simulink model "COM_test_gumstix"  (Simulink 8.6)
settings: Solver=FixedStepDiscrete  StartTime=0.0  StopTime=inf  FixedStep=ComMinSampleTime  RelTol=1e-3
values from neighbouring files (symbols this model uses):
  ComMinSampleTime = 1/200    (= 0.005)    [init_test_gumstix.m]
undefined symbols (not defined in the file or in its folder): BiasAcc, Gumstix, MPU6050, Tacc
undefined symbols (not defined in the file): g, m, Ts_AttitudeLoop, Ts_detector
libraries: custom_lib x25
settings Model: Creator=Kjenab  LastModifiedBy=valentin_riviere  ExtModeTrigDuration=10000
settings SolverCC: PositivePriorityOrder=on
settings DataIOCC: SaveFormat=StructureWithTime
settings OptimizationCC: InitFltsAndDblsToZero=on  OptimizeModelRefInitCode=on  LifeSpan=Inf  SimCompilerOptimization=on
settings DebuggingCC: SaveWithParameterizedLinksMsg=none  UnderspecifiedInitializationDetection=Simplified  MergeDetectMultiDrivingBlocksExec=error  FcnCallInpInsideContextMsg=UseLocalSettings
settings HardwareCC: ProdHWDeviceType=Generic->Unspecified (assume 32-bit Generic)
settings RTWCC: SystemTargetFile=ert.tlc  GenCodeOnly=on  GenerateMakefile=off  TemplateMakefile=ert_default_tmf  PostCodeGenCommand=packNGo(buildInfo, {'packType' 'hierarchical'})  Description=Embedded Coder  RTWCompilerOptimization=on
settings CodeAppCC: IgnoreCustomStorageClasses=off  CustomSymbolStrType=$N$R$M  InternalIdentifier=Classic
settings ERTTargetCC: MultiwordLength=2048  GenerateSampleERTMain=on  ERTCustomFileTemplate=example_file_process.tlc  ConvertIfToSwitch=off  SuppressUnreachableDefaultCases=off

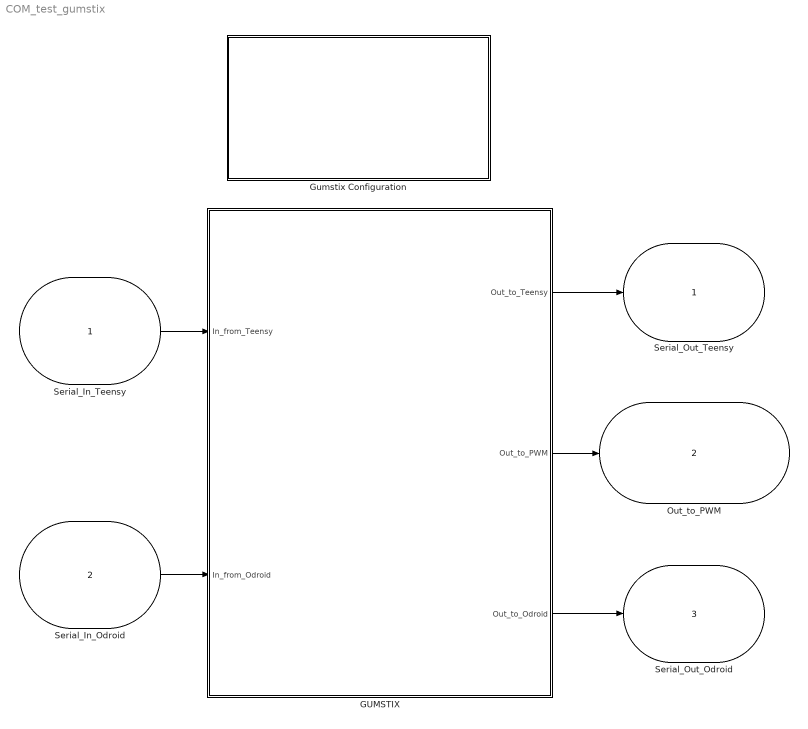
== system COM_test_gumstix ==
  Serial_In_Teensy : Inport  OutDataTypeStr=int16  PortDimensions=Gumstix.RS232.Reception(1).NbData  SampleTime=Gumstix.RS232.Reception(1).SampleTime  mask{RS232_NbData=27, RS232_DataType=int16, RS232_Port=/dev/ttyO0, RS232_BaudRate=115200, RS232_SampleTime=Ts_AttitudeLoop, RS232_BlockingReception=OFF (try to read the n data), RS232_BlockingTimeOut=0.001, RS232_StreamHeaderReception=1 byte, RS232_StreamHeaderValue=170, RS232_StartProtocol=SendStart -> WaitStart, RS232_StartTimeOut=100, RS232_StartStream=START, RS232_StopProtocol=None, RS232_StopTimeOut=100, RS232_StopStream=STOP}
      mask prompts: RS232_NbData "Number of Received Data"; RS232_DataType "RS232 Data Type"; RS232_Port "Serial Port"; RS232_BaudRate "BaudRate"; RS232_SampleTime "Reception Sample Time [s]"; RS232_BlockingReception "Blocking Reception"; RS232_BlockingTimeOut "Blocking Time Out [s]"; RS232_StreamHeaderReception "Stream Header"; RS232_StreamHeaderValue "Stream header value [0-255]"; RS232_StartProtocol "START Protocols"; RS232_StartTimeOut "Start Stream Waiting TimeOut [ms]"; RS232_StartStream "Start Message"; RS232_StopProtocol "STOP Protocols"; RS232_StopTimeOut "Stop Stream Waiting TimeOut [ms]"; RS232_StopStream "Stop Message"
      mask init:
      | for i=1:1:15
      |     ProcessRS232InportMask_COM(gcb, i);
      | end
      mask Callback RS232_NbData: ProcessRS232InportMask_COM(gcb, 1);
      mask TypeOptions RS232_DataType: double64 | float32 | int32 | unsigned int32 | int16 | unsigned int16 | char8 | unsigned char8
      mask Callback RS232_DataType: ProcessRS232InportMask_COM(gcb, 2);
      mask TypeOptions RS232_Port: /dev/ttyO0 | /dev/ttyO1 | /dev/ttyO2 | /dev/ttyO3 | /dev/ttyO4 | /dev/ttyO5 | /dev/ttyO6 | /dev/ttyO7 | /dev/ttyO8 | /dev/ttyO9 | /dev/ttyO10 | /dev/ttyO11 | /dev/ttyO12 | /dev/ttyO13 | /dev/ttyO14 | /dev/ttyO15 | /dev/ttyUSB0 | /dev/ttyUSB1
      mask Callback RS232_Port: ProcessRS232InportMask_COM(gcb, 3);
      mask TypeOptions RS232_BaudRate: 50 | 75 | 110 | 134 | 150 | 200 | 300 | 600 | 1200 | 1800 | 2400 | 4800 | 9600 | 19200 | 38400 | 57600 | 115200 | 230400 | 460800 | 576000 | 921600 | 1000000 | 1152000 | 1500000 | 2000000 | 2500000 | 3000000 | 3500000 | 4000000
      mask Callback RS232_BaudRate: ProcessRS232InportMask_COM(gcb, 4);
      mask Callback RS232_SampleTime: ProcessRS232InportMask_COM(gcb, 5);
      mask TypeOptions RS232_BlockingReception: ON (wait the n data) | OFF (try to read the n data)
      mask Callback RS232_BlockingReception: ProcessRS232InportMask_COM(gcb, 6);
      mask Callback RS232_BlockingTimeOut: ProcessRS232InportMask_COM(gcb, 7);
      mask TypeOptions RS232_StreamHeaderReception: None | 1 byte
      mask Callback RS232_StreamHeaderReception: ProcessRS232InportMask_COM(gcb, 8);
      mask Callback RS232_StreamHeaderValue: ProcessRS232InportMask_COM(gcb, 9);
      mask TypeOptions RS232_StartProtocol: WaitStart -> SendStart | SendStart -> WaitStart | None
      mask Callback RS232_StartProtocol: ProcessRS232InportMask_COM(gcb, 10);
      mask Callback RS232_StartTimeOut: ProcessRS232InportMask_COM(gcb, 11);
      mask Callback RS232_StartStream: ProcessRS232InportMask_COM(gcb, 12);
      mask TypeOptions RS232_StopProtocol: WaitStop -> SendStop | SendStop -> WaitStop | None
      mask Callback RS232_StopProtocol: ProcessRS232InportMask_COM(gcb, 13);
      mask Callback RS232_StopTimeOut: ProcessRS232InportMask_COM(gcb, 14);
      mask Callback RS232_StopStream: ProcessRS232InportMask_COM(gcb, 15);
      mask Display: Display_RS232_Reception_Block;
  Serial_In_Odroid : Inport  Port=2  OutDataTypeStr=uint8  PortDimensions=Gumstix.RS232.Reception(2).NbData  SampleTime=Gumstix.RS232.Reception(2).SampleTime  mask{RS232_NbData=28, RS232_DataType=unsigned char8, RS232_Port=/dev/ttyO2, RS232_BaudRate=115200, RS232_SampleTime=Ts_detector, RS232_BlockingReception=OFF (try to read the n data), RS232_BlockingTimeOut=0.001, RS232_StreamHeaderReception=1 byte, RS232_StreamHeaderValue=170, RS232_StartProtocol=SendStart -> WaitStart, RS232_StartTimeOut=100, RS232_StartStream=START, RS232_StopProtocol=None, RS232_StopTimeOut=100, RS232_StopStream=STOP}
      mask prompts: RS232_NbData "Number of Received Data"; RS232_DataType "RS232 Data Type"; RS232_Port "Serial Port"; RS232_BaudRate "BaudRate"; RS232_SampleTime "Reception Sample Time [s]"; RS232_BlockingReception "Blocking Reception"; RS232_BlockingTimeOut "Blocking Time Out [s]"; RS232_StreamHeaderReception "Stream Header"; RS232_StreamHeaderValue "Stream header value [0-255]"; RS232_StartProtocol "START Protocols"; RS232_StartTimeOut "Start Stream Waiting TimeOut [ms]"; RS232_StartStream "Start Message"; RS232_StopProtocol "STOP Protocols"; RS232_StopTimeOut "Stop Stream Waiting TimeOut [ms]"; RS232_StopStream "Stop Message"
      mask init:
      | for i=1:1:15
      |     ProcessRS232InportMask_COM(gcb, i);
      | end
      mask Callback RS232_NbData: ProcessRS232InportMask_COM(gcb, 1);
      mask TypeOptions RS232_DataType: double64 | float32 | int32 | unsigned int32 | int16 | unsigned int16 | char8 | unsigned char8
      mask Callback RS232_DataType: ProcessRS232InportMask_COM(gcb, 2);
      mask TypeOptions RS232_Port: /dev/ttyO0 | /dev/ttyO1 | /dev/ttyO2 | /dev/ttyO3 | /dev/ttyO4 | /dev/ttyO5 | /dev/ttyO6 | /dev/ttyO7 | /dev/ttyO8 | /dev/ttyO9 | /dev/ttyO10 | /dev/ttyO11 | /dev/ttyO12 | /dev/ttyO13 | /dev/ttyO14 | /dev/ttyO15 | /dev/ttyUSB0 | /dev/ttyUSB1
      mask Callback RS232_Port: ProcessRS232InportMask_COM(gcb, 3);
      mask TypeOptions RS232_BaudRate: 50 | 75 | 110 | 134 | 150 | 200 | 300 | 600 | 1200 | 1800 | 2400 | 4800 | 9600 | 19200 | 38400 | 57600 | 115200 | 230400 | 460800 | 576000 | 921600 | 1000000 | 1152000 | 1500000 | 2000000 | 2500000 | 3000000 | 3500000 | 4000000
      mask Callback RS232_BaudRate: ProcessRS232InportMask_COM(gcb, 4);
      mask Callback RS232_SampleTime: ProcessRS232InportMask_COM(gcb, 5);
      mask TypeOptions RS232_BlockingReception: ON (wait the n data) | OFF (try to read the n data)
      mask Callback RS232_BlockingReception: ProcessRS232InportMask_COM(gcb, 6);
      mask Callback RS232_BlockingTimeOut: ProcessRS232InportMask_COM(gcb, 7);
      mask TypeOptions RS232_StreamHeaderReception: None | 1 byte
      mask Callback RS232_StreamHeaderReception: ProcessRS232InportMask_COM(gcb, 8);
      mask Callback RS232_StreamHeaderValue: ProcessRS232InportMask_COM(gcb, 9);
      mask TypeOptions RS232_StartProtocol: WaitStart -> SendStart | SendStart -> WaitStart | None
      mask Callback RS232_StartProtocol: ProcessRS232InportMask_COM(gcb, 10);
      mask Callback RS232_StartTimeOut: ProcessRS232InportMask_COM(gcb, 11);
      mask Callback RS232_StartStream: ProcessRS232InportMask_COM(gcb, 12);
      mask TypeOptions RS232_StopProtocol: WaitStop -> SendStop | SendStop -> WaitStop | None
      mask Callback RS232_StopProtocol: ProcessRS232InportMask_COM(gcb, 13);
      mask Callback RS232_StopTimeOut: ProcessRS232InportMask_COM(gcb, 14);
      mask Callback RS232_StopStream: ProcessRS232InportMask_COM(gcb, 15);
      mask Display: Display_RS232_Reception_Block;
  GUMSTIX : Subsystem
  Gumstix Configuration : Subsystem  mask{TimeSynchro=Internal Clock, RS232_InterruptSource=/dev/ttyO0, UDP_InterruptSource=wlan0, PrintfMode=off, FprintfMode=off, TimeLoggerMode=off, PrintfTimeMode=off, FprintfTimeMode=off, TaskingMode=Multi-Tasking, SchedPolicy=SCHED_FIFO     (Real-Time Scheduler), MaxTaskPriority=95, RTsystem=PREEMPT-RT, TargetEndianess=Unspecified (default), TargetWordSize=32 bits (default)}
      mask prompts: TimeSynchro "Time Scheduler"; RS232_InterruptSource "RS232 Interrupt Source"; UDP_InterruptSource "UDP Interrupt Source"; PrintfMode "Verbose mode activated in the Gumstix console"; FprintfMode "Verbose mode logged in a file (onto Gumstix)"; TimeLoggerMode "Time logger mode activated (log time exec of each task)"; PrintfTimeMode "Execution time plotted in the Gumstix console"; FprintfTimeMode "Execution time logged in a file (onto Gumstix)"; TaskingMode "Tasking Mode"; SchedPolicy "Scheduler Policy"; MaxTaskPriority "Maximum Task Priority [1-99]"; RTsystem "RT system"; TargetEndianess "Target Endianess"; TargetWordSize "Target Word Size"
      mask init:
      | for i=1:1:14
      |     ProcessConfigMask_COM(gcb, i);
      | end
      mask TypeOptions TimeSynchro: RS232 Reception | Internal Clock | UDP Reception
      mask Callback TimeSynchro: ProcessConfigMask_COM(gcb, 1);
      mask TypeOptions RS232_InterruptSource: /dev/ttyS0 | /dev/ttyS1 | /dev/ttyS2 | /dev/ttyS3 | /dev/ttyO0 | /dev/ttyO1 | /dev/ttyO2 | /dev/ttyO3
      mask Callback RS232_InterruptSource: ProcessConfigMask_COM(gcb, 2);
      mask TypeOptions UDP_InterruptSource: wlan0 | eth0
      mask Callback UDP_InterruptSource: ProcessConfigMask_COM(gcb, 3);
      mask TypeOptions PrintfMode: off | on
      mask Callback PrintfMode: ProcessConfigMask_COM(gcb, 4);
      mask TypeOptions FprintfMode: off | on
      mask Callback FprintfMode: ProcessConfigMask_COM(gcb, 5);
      mask TypeOptions TimeLoggerMode: off | on
      mask Callback TimeLoggerMode: ProcessConfigMask_COM(gcb, 6);
      mask TypeOptions PrintfTimeMode: off | on
      mask Callback PrintfTimeMode: ProcessConfigMask_COM(gcb, 7);
      mask TypeOptions FprintfTimeMode: off | on
      mask Callback FprintfTimeMode: ProcessConfigMask_COM(gcb, 8);
      mask TypeOptions TaskingMode: Multi-Tasking | Single-Tasking
      mask Callback TaskingMode: ProcessConfigMask_COM(gcb, 9);
      mask TypeOptions SchedPolicy: SCHED_FIFO     (Real-Time Scheduler) | SCHED_RR        (Real-Time Scheduler) | SCHED_OTHER (NO Real-Time Scheduler)
      mask Callback SchedPolicy: ProcessConfigMask_COM(gcb, 10);
      mask Callback MaxTaskPriority: ProcessConfigMask_COM(gcb, 11);
      mask TypeOptions RTsystem: PREEMPT-RT | XENOMAI
      mask Callback RTsystem: ProcessConfigMask_COM(gcb, 12);
      mask TypeOptions TargetEndianess: Unspecified (default) | Little-Endian | Big-Endian
      mask Callback TargetEndianess: ProcessConfigMask_COM(gcb, 13);
      mask TypeOptions TargetWordSize: 32 bits (default) | 64 bits (LLP64) | 64 bits (LP64)
      mask Callback TargetWordSize: ProcessConfigMask_COM(gcb, 14);
      mask Display: image(imread('Configuration_v2.jpg'));
  Serial_Out_Teensy : Outport  OutDataTypeStr=int16  PortDimensions=Gumstix.RS232.Emission(1).NbData  SampleTime=Gumstix.RS232.Emission(1).SampleTime  mask{RS232_NbData=4, RS232_DataType=int16, RS232_Port=/dev/ttyO0, RS232_BaudRate=115200, RS232_SampleTime=Ts_AttitudeLoop, RS232_StreamHeaderReception=1 byte, RS232_StreamHeaderValue=170, RS232_StartProtocol=SendStart -> WaitStart, RS232_StartTimeOut=100, RS232_StartStream=START, RS232_StopProtocol=None, RS232_StopTimeOut=100, RS232_StopStream=STOP}
      mask prompts: RS232_NbData "Number of Sent Data"; RS232_DataType "RS232 Data Type"; RS232_Port "Serial Port"; RS232_BaudRate "BaudRate"; RS232_SampleTime "Sample Time [s]"; RS232_StreamHeaderReception "Stream Header"; RS232_StreamHeaderValue "Stream header value [0-255]"; RS232_StartProtocol "RS232 Start Protocol"; RS232_StartTimeOut "Start Stream Waiting TimeOut [ms]"; RS232_StartStream "Start Message"; RS232_StopProtocol "RS232 Stop Protocol"; RS232_StopTimeOut "Stop Stream Waiting TimeOut [ms]"; RS232_StopStream "Stop Message"
      mask init:
      | for i=1:1:13
      |     ProcessRS232OutportMask_COM(gcb, i);
      | end
      mask Callback RS232_NbData: ProcessRS232OutportMask_COM(gcb, 1);
      mask TypeOptions RS232_DataType: double64 | float32 | int32 | unsigned int32 | int16 | unsigned int16 | char8 | unsigned char8
      mask Callback RS232_DataType: ProcessRS232OutportMask_COM(gcb, 2);
      mask TypeOptions RS232_Port: /dev/ttyO0 | /dev/ttyO1 | /dev/ttyO2 | /dev/ttyO3 | /dev/ttyO4 | /dev/ttyO5 | /dev/ttyO6 | /dev/ttyO7 | /dev/ttyO8 | /dev/ttyO9 | /dev/ttyO10 | /dev/ttyO11 | /dev/ttyO12 | /dev/ttyO13 | /dev/ttyO14 | /dev/ttyO15 | /dev/ttyUSB0 | /dev/ttyUSB1
      mask Callback RS232_Port: ProcessRS232OutportMask_COM(gcb, 3);
      mask TypeOptions RS232_BaudRate: 50 | 75 | 110 | 134 | 150 | 200 | 300 | 600 | 1200 | 1800 | 2400 | 4800 | 9600 | 19200 | 38400 | 57600 | 115200 | 230400 | 460800 | 576000 | 921600 | 1000000 | 1152000 | 1500000 | 2000000 | 2500000 | 3000000 | 3500000 | 4000000
      mask Callback RS232_BaudRate: ProcessRS232OutportMask_COM(gcb, 4);
      mask Callback RS232_SampleTime: ProcessRS232OutportMask_COM(gcb, 5);
      mask TypeOptions RS232_StreamHeaderReception: None | 1 byte
      mask Callback RS232_StreamHeaderReception: ProcessRS232OutportMask_COM(gcb, 6);
      mask Callback RS232_StreamHeaderValue: ProcessRS232OutportMask_COM(gcb, 7);
      mask TypeOptions RS232_StartProtocol: WaitStart -> SendStart | SendStart -> WaitStart | None
      mask Callback RS232_StartProtocol: ProcessRS232OutportMask_COM(gcb, 8);
      mask Callback RS232_StartTimeOut: ProcessRS232OutportMask_COM(gcb, 9);
      mask Callback RS232_StartStream: ProcessRS232OutportMask_COM(gcb, 10);
      mask TypeOptions RS232_StopProtocol: WaitStop -> SendStop | SendStop -> WaitStop | None
      mask Callback RS232_StopProtocol: ProcessRS232OutportMask_COM(gcb, 11);
      mask Callback RS232_StopTimeOut: ProcessRS232OutportMask_COM(gcb, 12);
      mask Callback RS232_StopStream: ProcessRS232OutportMask_COM(gcb, 13);
      mask Display: Display_RS232_Emission_Block;
  Out_to_PWM : Outport  Port=2  OutDataTypeStr=uint16  PortDimensions=evalin('base', 'length(Gumstix.PWM.ActivePwm)')  SampleTime=evalin('base', 'Gumstix.PWM.SampleTime')  mask{TimersList=[8,11], PwmFrequency=333, PwmMode=DUTY_CYCLE Mode, ServoMin=10000, ServoMax=20000, PWM_DefaultValue=30, PWM_SampleTime=ComMinSampleTime, PWM_KeepAfterStop=on}
      mask prompts: TimersList "Active PWM (example: [8,9,10,11])"; PwmFrequency "PWM Frequency [Hz]"; PwmMode "PWM Mode"; ServoMin "Servo Min Value [tenth's of us]"; ServoMax "Servo Max Value [tenth's of us]"; PWM_DefaultValue "Default Pwm Value"; PWM_SampleTime "Refresh Sample Time [s]"; PWM_KeepAfterStop "Keep Default Pwm Value after program stop"
      mask init:
      | for i=1:1:8
      |     ProcessPWMmask_COM(gcb, i);
      | end
      mask Callback TimersList: ProcessPWMmask_COM(gcb, 1);
      mask Callback PwmFrequency: ProcessPWMmask_COM(gcb, 2);
      mask TypeOptions PwmMode: SERVO Mode | DUTY_CYCLE Mode
      mask Callback PwmMode: ProcessPWMmask_COM(gcb, 3);
      mask Callback ServoMin: ProcessPWMmask_COM(gcb, 4);
      mask Callback ServoMax: ProcessPWMmask_COM(gcb, 5);
      mask Callback PWM_DefaultValue: ProcessPWMmask_COM(gcb, 6);
      mask Callback PWM_SampleTime: ProcessPWMmask_COM(gcb, 7);
      mask Callback PWM_KeepAfterStop: ProcessPWMmask_COM(gcb, 8);
      mask Display: Display_PWM_Block;
  Serial_Out_Odroid : Outport  Port=3  OutDataTypeStr=uint8  PortDimensions=Gumstix.RS232.Emission(2).NbData  SampleTime=Gumstix.RS232.Emission(2).SampleTime  mask{RS232_NbData=48, RS232_DataType=unsigned char8, RS232_Port=/dev/ttyO2, RS232_BaudRate=115200, RS232_SampleTime=Ts_detector, RS232_StreamHeaderReception=1 byte, RS232_StreamHeaderValue=170, RS232_StartProtocol=SendStart -> WaitStart, RS232_StartTimeOut=100, RS232_StartStream=START, RS232_StopProtocol=None, RS232_StopTimeOut=100, RS232_StopStream=STOP}
      mask prompts: RS232_NbData "Number of Sent Data"; RS232_DataType "RS232 Data Type"; RS232_Port "Serial Port"; RS232_BaudRate "BaudRate"; RS232_SampleTime "Sample Time [s]"; RS232_StreamHeaderReception "Stream Header"; RS232_StreamHeaderValue "Stream header value [0-255]"; RS232_StartProtocol "RS232 Start Protocol"; RS232_StartTimeOut "Start Stream Waiting TimeOut [ms]"; RS232_StartStream "Start Message"; RS232_StopProtocol "RS232 Stop Protocol"; RS232_StopTimeOut "Stop Stream Waiting TimeOut [ms]"; RS232_StopStream "Stop Message"
      mask init:
      | for i=1:1:13
      |     ProcessRS232OutportMask_COM(gcb, i);
      | end
      mask Callback RS232_NbData: ProcessRS232OutportMask_COM(gcb, 1);
      mask TypeOptions RS232_DataType: double64 | float32 | int32 | unsigned int32 | int16 | unsigned int16 | char8 | unsigned char8
      mask Callback RS232_DataType: ProcessRS232OutportMask_COM(gcb, 2);
      mask TypeOptions RS232_Port: /dev/ttyO0 | /dev/ttyO1 | /dev/ttyO2 | /dev/ttyO3 | /dev/ttyO4 | /dev/ttyO5 | /dev/ttyO6 | /dev/ttyO7 | /dev/ttyO8 | /dev/ttyO9 | /dev/ttyO10 | /dev/ttyO11 | /dev/ttyO12 | /dev/ttyO13 | /dev/ttyO14 | /dev/ttyO15 | /dev/ttyUSB0 | /dev/ttyUSB1
      mask Callback RS232_Port: ProcessRS232OutportMask_COM(gcb, 3);
      mask TypeOptions RS232_BaudRate: 50 | 75 | 110 | 134 | 150 | 200 | 300 | 600 | 1200 | 1800 | 2400 | 4800 | 9600 | 19200 | 38400 | 57600 | 115200 | 230400 | 460800 | 576000 | 921600 | 1000000 | 1152000 | 1500000 | 2000000 | 2500000 | 3000000 | 3500000 | 4000000
      mask Callback RS232_BaudRate: ProcessRS232OutportMask_COM(gcb, 4);
      mask Callback RS232_SampleTime: ProcessRS232OutportMask_COM(gcb, 5);
      mask TypeOptions RS232_StreamHeaderReception: None | 1 byte
      mask Callback RS232_StreamHeaderReception: ProcessRS232OutportMask_COM(gcb, 6);
      mask Callback RS232_StreamHeaderValue: ProcessRS232OutportMask_COM(gcb, 7);
      mask TypeOptions RS232_StartProtocol: WaitStart -> SendStart | SendStart -> WaitStart | None
      mask Callback RS232_StartProtocol: ProcessRS232OutportMask_COM(gcb, 8);
      mask Callback RS232_StartTimeOut: ProcessRS232OutportMask_COM(gcb, 9);
      mask Callback RS232_StartStream: ProcessRS232OutportMask_COM(gcb, 10);
      mask TypeOptions RS232_StopProtocol: WaitStop -> SendStop | SendStop -> WaitStop | None
      mask Callback RS232_StopProtocol: ProcessRS232OutportMask_COM(gcb, 11);
      mask Callback RS232_StopTimeOut: ProcessRS232OutportMask_COM(gcb, 12);
      mask Callback RS232_StopStream: ProcessRS232OutportMask_COM(gcb, 13);
      mask Display: Display_RS232_Emission_Block;
  wires:
  Serial_In_Teensy/1 -> GUMSTIX/1(In_from_Teensy)
  GUMSTIX/1(Out_to_Teensy) -> Serial_Out_Teensy/1
  GUMSTIX/2(Out_to_PWM) -> Out_to_PWM/1
  Serial_In_Odroid/1 -> GUMSTIX/2(In_from_Odroid)
  GUMSTIX/3(Out_to_Odroid) -> Serial_Out_Odroid/1

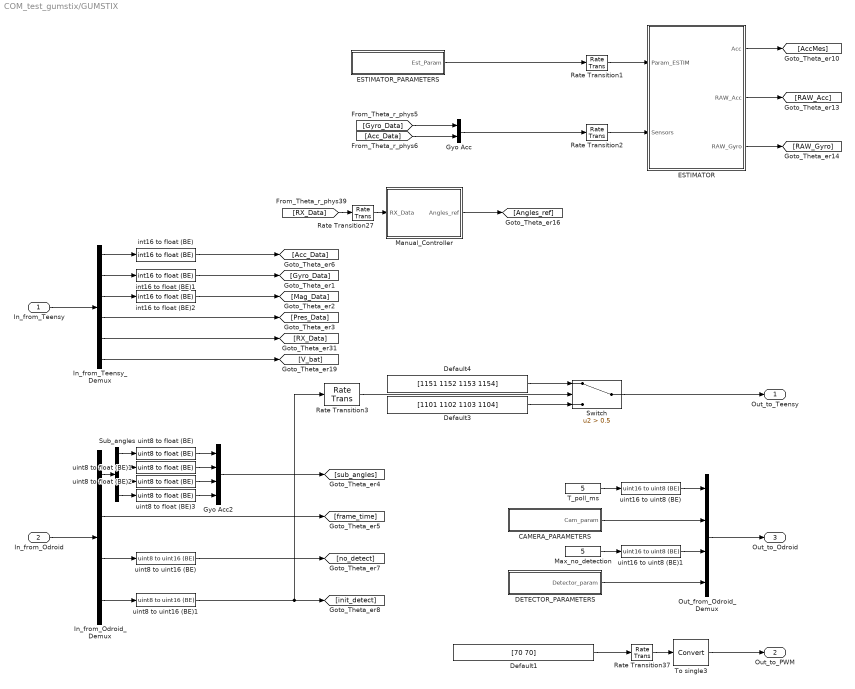
== system COM_test_gumstix/GUMSTIX ==
  In_from_Teensy : Inport
  In_from_Odroid : Inport  Port=2
  CAMERA_PARAMETERS : Subsystem
  DETECTOR_PARAMETERS : Subsystem
  Default1 : Constant  Value=[70 70]  OutDataTypeStr=Inherit: Inherit via back propagation  SampleTime=-1
  Default3 : Constant  Value=[1101 1102 1103 1104]  OutDataTypeStr=Inherit: Inherit via back propagation  SampleTime=-1
  Default4 : Constant  Value=[1151 1152 1153 1154]  OutDataTypeStr=Inherit: Inherit via back propagation  SampleTime=-1
  ESTIMATOR : Subsystem
  ESTIMATOR_PARAMETERS : Subsystem
  Gyo Acc : Mux  Inputs=2
  Gyo Acc2 : Mux
  In_from_Odroid_Demux : Demux  Outputs=[16 8 2 2]
  In_from_Teensy_Demux : Demux  Outputs=[6 6 6 4 4 1]
  Manual_Controller : Subsystem
  Max_no_detection : Constant  Value=5  OutDataTypeStr=Inherit: Inherit via back propagation  SampleTime=-1
  Out_from_Odroid_Demux : Mux  Inputs=[2 24 2 20]
  Rate Transition1 : RateTransition  Deterministic=off  OutPortSampleTime=Ts_AttitudeLoop
  Rate Transition2 : RateTransition  Deterministic=off  OutPortSampleTime=Ts_AttitudeLoop
  Rate Transition27 : RateTransition  Deterministic=off  OutPortSampleTime=Ts_PositionLoop
  Rate Transition3 : RateTransition  Deterministic=off
  Rate Transition37 : RateTransition  Deterministic=off
  Sub_angles : Demux
  Switch : Switch  Criteria=u2 > Threshold  Threshold=0.5
  T_poll_ms : Constant  Value=5  OutDataTypeStr=Inherit: Inherit via back propagation  SampleTime=-1
  To single3 : DataTypeConversion  RndMeth=Nearest
  int16 to float (BE) : custom_lib/CONVERTERS/int16 to float (BE)
  int16 to float (BE)1 : custom_lib/CONVERTERS/int16 to float (BE)
  int16 to float (BE)2 : custom_lib/CONVERTERS/int16 to float (BE)
  uint16 to uint8 (BE) : custom_lib/CONVERTERS/uint16 to uint8 (BE)
  uint16 to uint8 (BE)1 : custom_lib/CONVERTERS/uint16 to uint8 (BE)
  uint8 to float (BE){,1..3} (4 alike) : custom_lib/CONVERTERS/uint8 to float (BE)
  uint8 to uint16 (BE) : custom_lib/CONVERTERS/uint8 to uint16 (BE)
  uint8 to uint16 (BE)1 : custom_lib/CONVERTERS/uint8 to uint16 (BE)
  Out_to_Teensy : Outport
  Out_to_PWM : Outport  Port=2
  Out_to_Odroid : Outport  Port=3
  wires:
  In_from_Teensy_Demux/1 -> int16 to float (BE)/1
  In_from_Teensy/1 -> In_from_Teensy_Demux/1
  [Gyro_Data] -> Gyo Acc/1
  [Acc_Data] -> Gyo Acc/2
  [RX_Data] -> Rate Transition27/1
  ESTIMATOR_PARAMETERS/1(Est_Param) -> Rate Transition1/1
  In_from_Teensy_Demux/2 -> int16 to float (BE)1/1
  Manual_Controller/1(Angles_ref) -> [Angles_ref]
  Rate Transition27/1 -> Manual_Controller/1(RX_Data)
  Rate Transition1/1 -> ESTIMATOR/1(Param_ESTIM)
  Rate Transition2/1 -> ESTIMATOR/2(Sensors)
  ESTIMATOR/1(Acc) -> [AccMes]
  ESTIMATOR/2(RAW_Acc) -> [RAW_Acc]
  ESTIMATOR/3(RAW_Gyro) -> [RAW_Gyro]
  Default1/1 -> Rate Transition37/1
  Rate Transition37/1 -> To single3/1
  To single3/1 -> Out_to_PWM/1
  In_from_Teensy_Demux/3 -> int16 to float (BE)2/1
  In_from_Teensy_Demux/5 -> [RX_Data]
  In_from_Teensy_Demux/6 -> [V_bat]
  int16 to float (BE)/1 -> [Acc_Data]
  int16 to float (BE)1/1 -> [Gyro_Data]
  int16 to float (BE)2/1 -> [Mag_Data]
  In_from_Teensy_Demux/4 -> [Pres_Data]
  Gyo Acc/1 -> Rate Transition2/1
  In_from_Odroid/1 -> In_from_Odroid_Demux/1
  In_from_Odroid_Demux/1 -> Sub_angles/1
  Sub_angles/1 -> uint8 to float (BE)/1
  Sub_angles/2 -> uint8 to float (BE)1/1
  Sub_angles/3 -> uint8 to float (BE)2/1
  Sub_angles/4 -> uint8 to float (BE)3/1
  uint8 to float (BE)/1 -> Gyo Acc2/1
  uint8 to float (BE)1/1 -> Gyo Acc2/2
  uint8 to float (BE)2/1 -> Gyo Acc2/3
  uint8 to float (BE)3/1 -> Gyo Acc2/4
  Gyo Acc2/1 -> [sub_angles]
  In_from_Odroid_Demux/3 -> uint8 to uint16 (BE)/1
  In_from_Odroid_Demux/4 -> uint8 to uint16 (BE)1/1
  Out_from_Odroid_Demux/1 -> Out_to_Odroid/1
  T_poll_ms/1 -> uint16 to uint8 (BE)/1
  DETECTOR_PARAMETERS/1(Detector_param) -> Out_from_Odroid_Demux/4
  CAMERA_PARAMETERS/1(Cam_param) -> Out_from_Odroid_Demux/2
  uint16 to uint8 (BE)/1 -> Out_from_Odroid_Demux/1
  Max_no_detection/1 -> uint16 to uint8 (BE)1/1
  In_from_Odroid_Demux/2 -> [frame_time]
  Default4/1 -> Switch/1
  Default3/1 -> Switch/3
  Switch/1 -> Out_to_Teensy/1
  Rate Transition3/1 -> Switch/2
  uint16 to uint8 (BE)1/1 -> Out_from_Odroid_Demux/3
  uint8 to uint16 (BE)1/1 -> Rate Transition3/1, [init_detect]
  uint8 to uint16 (BE)/1 -> [no_detect]

== system COM_test_gumstix/Gumstix Configuration ==

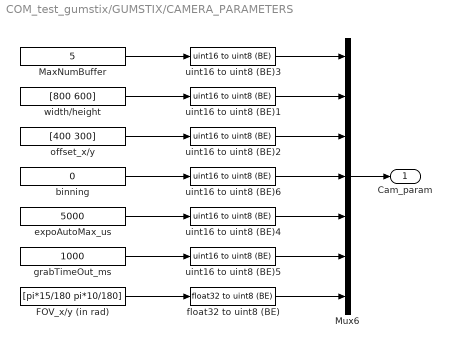
== system COM_test_gumstix/GUMSTIX/CAMERA_PARAMETERS ==
  FOV_x/y (in rad) : Constant  Value=[pi*15/180 pi*10/180]  OutDataTypeStr=Inherit: Inherit via back propagation  SampleTime=-1
  MaxNumBuffer : Constant  Value=5  OutDataTypeStr=Inherit: Inherit via back propagation  SampleTime=-1
  Mux6 : Mux  Inputs=[2 4 4 2 2 2 8]
  binning : Constant  Value=0  OutDataTypeStr=Inherit: Inherit via back propagation  SampleTime=-1
  expoAutoMax_us : Constant  Value=5000  OutDataTypeStr=Inherit: Inherit via back propagation  SampleTime=-1
  float32 to uint8 (BE) : custom_lib/CONVERTERS/float32 to uint8 (BE)
  grabTimeOut_ms : Constant  Value=1000  OutDataTypeStr=Inherit: Inherit via back propagation  SampleTime=-1
  offset_x/y : Constant  Value=[400 300]  OutDataTypeStr=Inherit: Inherit via back propagation  SampleTime=-1
  uint16 to uint8 (BE){1..6} (6 alike) : custom_lib/CONVERTERS/uint16 to uint8 (BE)
  width/height : Constant  Value=[800 600]  OutDataTypeStr=Inherit: Inherit via back propagation  SampleTime=-1
  Cam_param : Outport
  wires:
  width/height/1 -> uint16 to uint8 (BE)1/1
  offset_x/y/1 -> uint16 to uint8 (BE)2/1
  Mux6/1 -> Cam_param/1
  expoAutoMax_us/1 -> uint16 to uint8 (BE)4/1
  grabTimeOut_ms/1 -> uint16 to uint8 (BE)5/1
  FOV_x/y (in rad)/1 -> float32 to uint8 (BE)/1
  float32 to uint8 (BE)/1 -> Mux6/7
  MaxNumBuffer/1 -> uint16 to uint8 (BE)3/1
  uint16 to uint8 (BE)1/1 -> Mux6/2
  uint16 to uint8 (BE)2/1 -> Mux6/3
  binning/1 -> uint16 to uint8 (BE)6/1
  uint16 to uint8 (BE)4/1 -> Mux6/5
  uint16 to uint8 (BE)5/1 -> Mux6/6
  uint16 to uint8 (BE)3/1 -> Mux6/1
  uint16 to uint8 (BE)6/1 -> Mux6/4

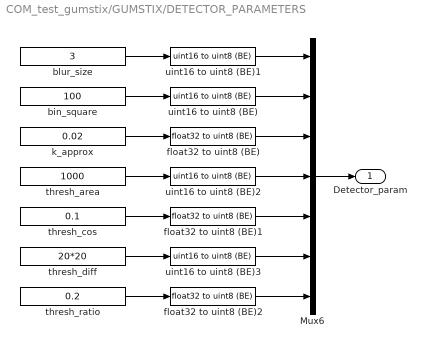
== system COM_test_gumstix/GUMSTIX/DETECTOR_PARAMETERS ==
  Mux6 : Mux  Inputs=[2 2 4 2 4 2 4]
  bin_square : Constant  Value=100  OutDataTypeStr=Inherit: Inherit via back propagation  SampleTime=-1
  blur_size : Constant  Value=3  OutDataTypeStr=Inherit: Inherit via back propagation  SampleTime=-1
  float32 to uint8 (BE) : custom_lib/CONVERTERS/float32 to uint8 (BE)
  float32 to uint8 (BE)1 : custom_lib/CONVERTERS/float32 to uint8 (BE)
  float32 to uint8 (BE)2 : custom_lib/CONVERTERS/float32 to uint8 (BE)
  k_approx : Constant  Value=0.02  OutDataTypeStr=Inherit: Inherit via back propagation  SampleTime=-1
  thresh_area : Constant  Value=1000  OutDataTypeStr=Inherit: Inherit via back propagation  SampleTime=-1
  thresh_cos : Constant  Value=0.1  OutDataTypeStr=Inherit: Inherit via back propagation  SampleTime=-1
  thresh_diff : Constant  Value=20*20  OutDataTypeStr=Inherit: Inherit via back propagation  SampleTime=-1
  thresh_ratio : Constant  Value=0.2  OutDataTypeStr=Inherit: Inherit via back propagation  SampleTime=-1
  uint16 to uint8 (BE){,1..3} (4 alike) : custom_lib/CONVERTERS/uint16 to uint8 (BE)
  Detector_param : Outport
  wires:
  Mux6/1 -> Detector_param/1
  thresh_ratio/1 -> float32 to uint8 (BE)2/1
  k_approx/1 -> float32 to uint8 (BE)/1
  thresh_area/1 -> uint16 to uint8 (BE)2/1
  thresh_cos/1 -> float32 to uint8 (BE)1/1
  thresh_diff/1 -> uint16 to uint8 (BE)3/1
  float32 to uint8 (BE)/1 -> Mux6/3
  float32 to uint8 (BE)1/1 -> Mux6/5
  float32 to uint8 (BE)2/1 -> Mux6/7
  blur_size/1 -> uint16 to uint8 (BE)1/1
  bin_square/1 -> uint16 to uint8 (BE)/1
  uint16 to uint8 (BE)2/1 -> Mux6/4
  uint16 to uint8 (BE)3/1 -> Mux6/6
  uint16 to uint8 (BE)1/1 -> Mux6/1
  uint16 to uint8 (BE)/1 -> Mux6/2

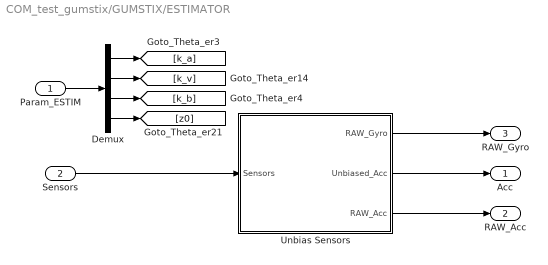
== system COM_test_gumstix/GUMSTIX/ESTIMATOR ==
  Param_ESTIM : Inport
  Sensors : Inport  Port=2
  Demux : Demux  Outputs=[3; 3; 3; 1]
  Unbias Sensors : Subsystem
  Acc : Outport
  RAW_Acc : Outport  Port=2
  RAW_Gyro : Outport  Port=3
  wires:
  Sensors/1 -> Unbias Sensors/1(Sensors)
  Unbias Sensors/2(Unbiased_Acc) -> Acc/1
  Unbias Sensors/1(RAW_Gyro) -> RAW_Gyro/1
  Param_ESTIM/1 -> Demux/1
  Demux/1 -> [k_a]
  Demux/2 -> [k_v]
  Demux/3 -> [k_b]
  Demux/4 -> [z0]
  Unbias Sensors/3(RAW_Acc) -> RAW_Acc/1

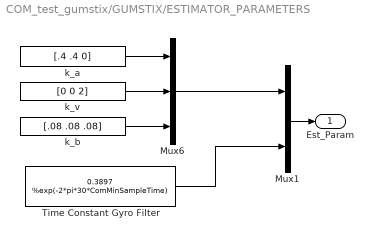
== system COM_test_gumstix/GUMSTIX/ESTIMATOR_PARAMETERS ==
  Mux1 : Mux  Inputs=2
  Mux6 : Mux  Inputs=3
  Time Constant Gyro Filter : Constant  Value=0.3897 %exp(-2*pi*30*ComMinSampleTime)  OutDataTypeStr=Inherit: Inherit via back propagation  SampleTime=-1
  k_a : Constant  Value=[.4 .4 0]  OutDataTypeStr=Inherit: Inherit via back propagation  SampleTime=-1
  k_b : Constant  Value=[.08 .08 .08]  OutDataTypeStr=Inherit: Inherit via back propagation  SampleTime=-1
  k_v : Constant  Value=[0 0 2]  OutDataTypeStr=Inherit: Inherit via back propagation  SampleTime=-1
  Est_Param : Outport
  wires:
  k_a/1 -> Mux6/1
  k_b/1 -> Mux6/3
  k_v/1 -> Mux6/2
  Mux6/1 -> Mux1/1
  Time Constant Gyro Filter/1 -> Mux1/2
  Mux1/1 -> Est_Param/1

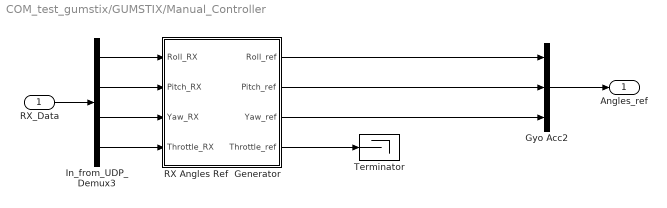
== system COM_test_gumstix/GUMSTIX/Manual_Controller ==
  RX_Data : Inport
  Gyo Acc2 : Mux  Inputs=[1 1 1]
  In_from_UDP_Demux3 : Demux  Outputs=[1 1 1 1]
  RX Angles Ref  Generator : Subsystem
  Terminator : Terminator
  Angles_ref : Outport
  wires:
  RX Angles Ref  Generator/1(Roll_ref) -> Gyo Acc2/1
  RX Angles Ref  Generator/2(Pitch_ref) -> Gyo Acc2/2
  RX Angles Ref  Generator/3(Yaw_ref) -> Gyo Acc2/3
  In_from_UDP_Demux3/1 -> RX Angles Ref  Generator/1(Roll_RX)
  In_from_UDP_Demux3/2 -> RX Angles Ref  Generator/2(Pitch_RX)
  In_from_UDP_Demux3/3 -> RX Angles Ref  Generator/3(Yaw_RX)
  In_from_UDP_Demux3/4 -> RX Angles Ref  Generator/4(Throttle_RX)
  RX_Data/1 -> In_from_UDP_Demux3/1
  Gyo Acc2/1 -> Angles_ref/1
  RX Angles Ref  Generator/4(Throttle_ref) -> Terminator/1

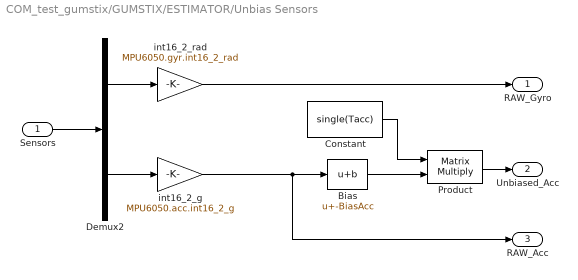
== system COM_test_gumstix/GUMSTIX/ESTIMATOR/Unbias Sensors ==
  Sensors : Inport
  Bias : Bias  Bias=-BiasAcc
  Constant : Constant  Value=single(Tacc)
  Demux2 : Demux  Outputs=[3 3]
  Product : Product  Multiplication=Matrix(*)  RndMeth=Zero
  int16_2_g : Gain  Gain=MPU6050.acc.int16_2_g  OutDataTypeStr=Inherit: Same as input
  int16_2_rad : Gain  Gain=MPU6050.gyr.int16_2_rad  OutDataTypeStr=Inherit: Same as input
  RAW_Gyro : Outport
  Unbiased_Acc : Outport  Port=2
  RAW_Acc : Outport  Port=3
  wires:
  Sensors/1 -> Demux2/1
  int16_2_g/1 -> RAW_Acc/1, Bias/1
  Demux2/1 -> int16_2_rad/1
  int16_2_rad/1 -> RAW_Gyro/1
  Demux2/2 -> int16_2_g/1
  Bias/1 -> Product/2
  Constant/1 -> Product/1
  Product/1 -> Unbiased_Acc/1

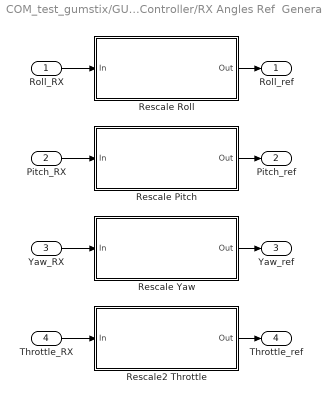
== system COM_test_gumstix/GUMSTIX/Manual_Controller/RX Angles Ref  Generator ==
  Roll_RX : Inport
  Pitch_RX : Inport  Port=2
  Yaw_RX : Inport  Port=3
  Throttle_RX : Inport  Port=4
  Rescale Pitch : Subsystem  mask{MinInput=1000, MaxInput=2000, DeadZone=10, MinOutput=-20*pi/180, MaxOutput=20*pi/180, G_Scale=0, BiasScale=0}
      mask prompts: MinInput "Minimum Input"; MaxInput "Maximum Input"; DeadZone "Dead Zone"; MinOutput "Minimum Output"; MaxOutput "Maximum Output"; BiasScale "Bias_Scale"
      mask init:
      | Gscale = (MaxOutput-MinOutput)/(MaxInput-MinInput-2*DeadZone);
      | Bias_Scale = MinInput+(MaxInput-MinInput)/2;
  Rescale Roll : Subsystem  mask{MinInput=1000, MaxInput=2000, DeadZone=10, MinOutput=-20*pi/180, MaxOutput=20*pi/180, G_Scale=0, BiasScale=0}
      mask prompts: MinInput "Minimum Input"; MaxInput "Maximum Input"; DeadZone "Dead Zone"; MinOutput "Minimum Output"; MaxOutput "Maximum Output"; BiasScale "Bias_Scale"
      mask init:
      | Gscale = (MaxOutput-MinOutput)/(MaxInput-MinInput-2*DeadZone);
      | Bias_Scale = MinInput+(MaxInput-MinInput)/2;
  Rescale Yaw : Subsystem  mask{MinInput=1000, MaxInput=2000, DeadZone=10, MinOutput=-30*pi/180, MaxOutput=30*pi/180, G_Scale=0, BiasScale=0}
      mask prompts: MinInput "Minimum Input"; MaxInput "Maximum Input"; DeadZone "Dead Zone"; MinOutput "Minimum Output"; MaxOutput "Maximum Output"; BiasScale "Bias_Scale"
      mask init:
      | Gscale = (MaxOutput-MinOutput)/(MaxInput-MinInput-2*DeadZone);
      | Bias_Scale = MinInput+(MaxInput-MinInput)/2;
  Rescale2 Throttle : Subsystem  mask{MinInput=1000, MaxInput=2000, MinOutput=0*m*g, MaxOutput=1.3*m*g, G_Scale=0}
      mask prompts: MinInput "Minimum Input"; MaxInput "Maximum Input"; MinOutput "Minimum Output"; MaxOutput "Maximum Output"
      mask init:
      | Gscale = (MaxOutput-MinOutput)/(MaxInput-MinInput);
  Roll_ref : Outport
  Pitch_ref : Outport  Port=2
  Yaw_ref : Outport  Port=3
  Throttle_ref : Outport  Port=4
  wires:
  Roll_RX/1 -> Rescale Roll/1(In)
  Pitch_RX/1 -> Rescale Pitch/1(In)
  Yaw_RX/1 -> Rescale Yaw/1(In)
  Rescale Roll/1(Out) -> Roll_ref/1
  Rescale Pitch/1(Out) -> Pitch_ref/1
  Rescale Yaw/1(Out) -> Yaw_ref/1
  Throttle_RX/1 -> Rescale2 Throttle/1(In)
  Rescale2 Throttle/1(Out) -> Throttle_ref/1

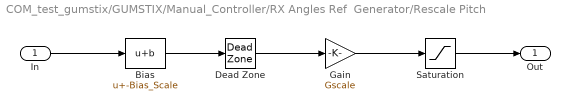
== system COM_test_gumstix/GUMSTIX/Manual_Controller/RX Angles Ref  Generator/Rescale Pitch ==
  In : Inport
  Bias : Bias  Bias=-Bias_Scale
  Dead Zone : DeadZone  LowerValue=-DeadZone  UpperValue=DeadZone  SaturateOnIntegerOverflow=on
  Gain : Gain  Gain=Gscale  OutDataTypeStr=Inherit: Inherit via back propagation
  Saturation : Saturate  UpperLimit=MaxOutput  LowerLimit=MinOutput
  Out : Outport
  wires:
  Bias/1 -> Dead Zone/1
  In/1 -> Bias/1
  Dead Zone/1 -> Gain/1
  Saturation/1 -> Out/1
  Gain/1 -> Saturation/1

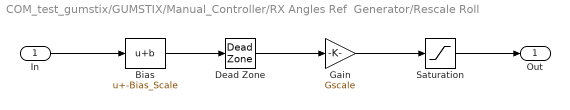
== system COM_test_gumstix/GUMSTIX/Manual_Controller/RX Angles Ref  Generator/Rescale Roll ==
  In : Inport
  Bias : Bias  Bias=-Bias_Scale
  Dead Zone : DeadZone  LowerValue=-DeadZone  UpperValue=DeadZone  SaturateOnIntegerOverflow=on
  Gain : Gain  Gain=Gscale  OutDataTypeStr=Inherit: Inherit via back propagation
  Saturation : Saturate  UpperLimit=MaxOutput  LowerLimit=MinOutput
  Out : Outport
  wires:
  Gain/1 -> Saturation/1
  Saturation/1 -> Out/1
  Dead Zone/1 -> Gain/1
  In/1 -> Bias/1
  Bias/1 -> Dead Zone/1

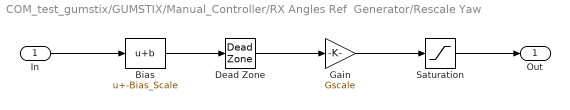
== system COM_test_gumstix/GUMSTIX/Manual_Controller/RX Angles Ref  Generator/Rescale Yaw ==
  In : Inport
  Bias : Bias  Bias=-Bias_Scale
  Dead Zone : DeadZone  LowerValue=-DeadZone  UpperValue=DeadZone  SaturateOnIntegerOverflow=on
  Gain : Gain  Gain=Gscale  OutDataTypeStr=Inherit: Inherit via back propagation
  Saturation : Saturate  UpperLimit=MaxOutput  LowerLimit=MinOutput
  Out : Outport
  wires:
  Gain/1 -> Saturation/1
  Saturation/1 -> Out/1
  Dead Zone/1 -> Gain/1
  In/1 -> Bias/1
  Bias/1 -> Dead Zone/1

== system COM_test_gumstix/GUMSTIX/Manual_Controller/RX Angles Ref  Generator/Rescale2 Throttle ==
  In : Inport
  Bias : Bias  Bias=-MinInput
  Gain : Gain  Gain=Gscale  OutDataTypeStr=Inherit: Inherit via back propagation
  Saturation : Saturate  UpperLimit=MaxOutput  LowerLimit=MinOutput
  Out : Outport
  wires:
  Bias/1 -> Gain/1
  In/1 -> Bias/1
  Saturation/1 -> Out/1
  Gain/1 -> Saturation/1
